simulink model "adjointmodel"  (Simulink 7.7)
settings: Solver=ode45  StartTime=0.0  StopTime=10.0  RelTol=1e-3
values from neighbouring files (symbols this model uses):
  tstep = 0.1    [lab8.m]
libraries: simulink x1
settings Model: Creator=student  LastModifiedBy=mestan
settings DataIOCC: LimitDataPoints=off

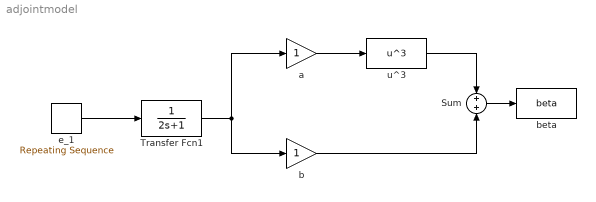
== system adjointmodel ==
  Sum : Sum  Inputs=+|+
  Transfer Fcn1 : TransferFcn  Denominator=[2 1]
  a : Gain
  b : Gain
  beta : ToWorkspace  VariableName=beta  SampleTime=tstep  SaveFormat=Array
  e_1 : simulink/Sources/Repeating Sequence  SystemSampleTime=-1  rep_seq_t=t  rep_seq_y=e_1
  u^3 : Fcn  Expr=u^3
  wires:
  e_1/1 -> Transfer Fcn1/1
  Transfer Fcn1/1 -> a/1, b/1
  b/1 -> Sum/2
  Sum/1 -> beta/1
  u^3/1 -> Sum/1
  a/1 -> u^3/1
